simulink model "verify_VDIHeatExchanger_mdl"  (R2018b)
settings: Solver=ode45  StartTime=0.0  StopTime=3600  MaxStep=600  RelTol=1e-3  EnableMultiTasking=on
undefined symbols (not defined in the file or in its folder): path_carnot
libraries: carnot x5
settings Model: Creator=drhf  LastModifiedBy=oetringer
settings DataIOCC: LimitDataPoints=on  SaveFormat=Array  SignalLoggingSaveFormat=ModelDataLogs  SignalLogging=off
settings OptimizationCC: ExpressionDepthLimit=2147483647  LifeSpan=inf
settings DebuggingCC: UnderspecifiedInitializationDetection=Classic  MergeDetectMultiDrivingBlocksExec=none  SolverPrmCheckMsg=warning  FcnCallInpInsideContextMsg=warning  StateNameClashWarn=warning  SFUnexpectedBacktrackingDiag=warning  SFNoUnconditionalDefaultTransitionDiag=warning  SFExecutionAtInitializationDiag=none
settings HardwareCC: ProdBitPerPointer=32  ProdBitPerSizeT=32  ProdBitPerPtrDiffT=32  ProdLargestAtomicFloat=None  ProdIntDivRoundTo=Undefined  ProdEndianess=Unspecified  ProdWordSize=32  ProdHWDeviceType=32-bit Generic
settings ModelReferenceCC: PropagateSignalLabelsOutOfModel=off
settings SFSimCC: SimUseLocalCustomCode=off
settings RTWCC: RTWUseLocalCustomCode=off
settings CodeAppCC: StateflowObjectComments=on
settings GRTTargetCC: TargetLangStandard=C89/C90 (ANSI)  GeneratePreprocessorConditionals=Disable all  CombineOutputUpdateFcns=off  GRTInterface=on
settings ConfigComp: CovMetricSettings=dw  CovHtmlReporting=on  CovSaveCumulativeToWorkspaceVar=on  CovSaveSingleToWorkspaceVar=on  CovExternalEMLEnable=off

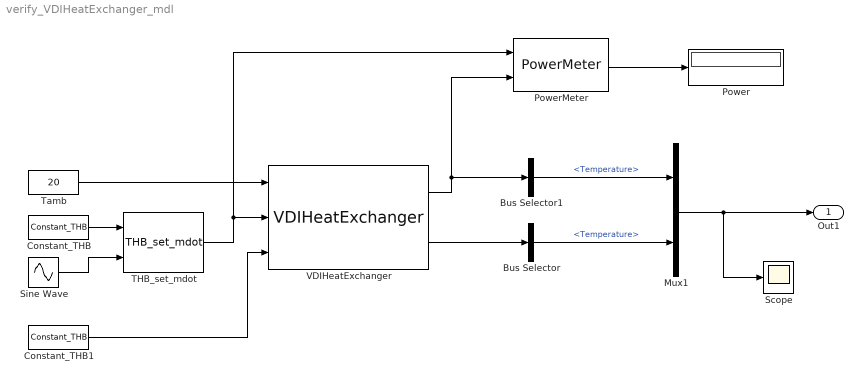
== system verify_VDIHeatExchanger_mdl ==
  Bus Selector : BusSelector  OutputSignals=Temperature
  Bus Selector1 : BusSelector  OutputSignals=Temperature
  Constant_THB : carnot/Source/Simple/Constant_THB  t=40  mdot=50/3600  p=1e5  mID=No Pressure Drop  fluid=Water  mix=0  mix2=0  mix3=0  dia=0.02  hgt=0
  Constant_THB1 : carnot/Source/Simple/Constant_THB  t=10  mdot=500/3600  p=1e5  mID=No Pressure Drop  fluid=Water  mix=0  mix2=0  mix3=0  dia=0.02  hgt=0
  Mux1 : Mux  Inputs=2
  Power : Display
  PowerMeter : carnot/Control/PowerMeter
  Scope : Scope
  Sine Wave : Sin  Amplitude=500/3600  Bias=400/3600  Frequency=2*pi/3600  SampleTime=0
  THB_set_mdot : carnot/Source/Simple/THB_set_mdot
  Tamb : Constant  Value=20
  VDIHeatExchanger : carnot/Source/Heat_Exchanger/VDIHeatExchanger  t0=20  PathName=fullfile(path_carnot('intlibsl'), 'Source', 'Heat_Exchanger', 'VDIHeatExchanger', 'parameter_set')  FileName='<user defined>'  userPath=off  userParam=on  flowtype=1  a=0  b=0  c=0  d=0  ua0=2000  uahot=[0.04 0]  uacold=[0.04 0]  ualoss=0  cap=10000  linh=20  quah=10  linc=20  quac=10
  Out1 : Outport  SampleTime=120
  wires:
  THB_set_mdot/1 -> VDIHeatExchanger/2, PowerMeter/1
  PowerMeter/1 -> Power/1
  VDIHeatExchanger/1 -> Bus Selector1/1, PowerMeter/2
  Constant_THB/1 -> THB_set_mdot/1
  Sine Wave/1 -> THB_set_mdot/2
  Constant_THB1/1 -> VDIHeatExchanger/3
  Tamb/1 -> VDIHeatExchanger/1
  VDIHeatExchanger/2 -> Bus Selector/1
  Bus Selector/1 -> Mux1/2  "<Temperature>"
  Bus Selector1/1 -> Mux1/1  "<Temperature>"
  Mux1/1 -> Out1/1, Scope/1
